simulink model "Rotational_to_linear"  (R2019a)
settings: Solver=VariableStepAuto  StartTime=0.0  StopTime=10  RelTol=1e-3
undefined symbols (not defined in the file): k_A, k_B, sigma_A, sigma_B
libraries: simulink x4
settings Model: Creator=wsimpson  LastModifiedBy=wsimpson

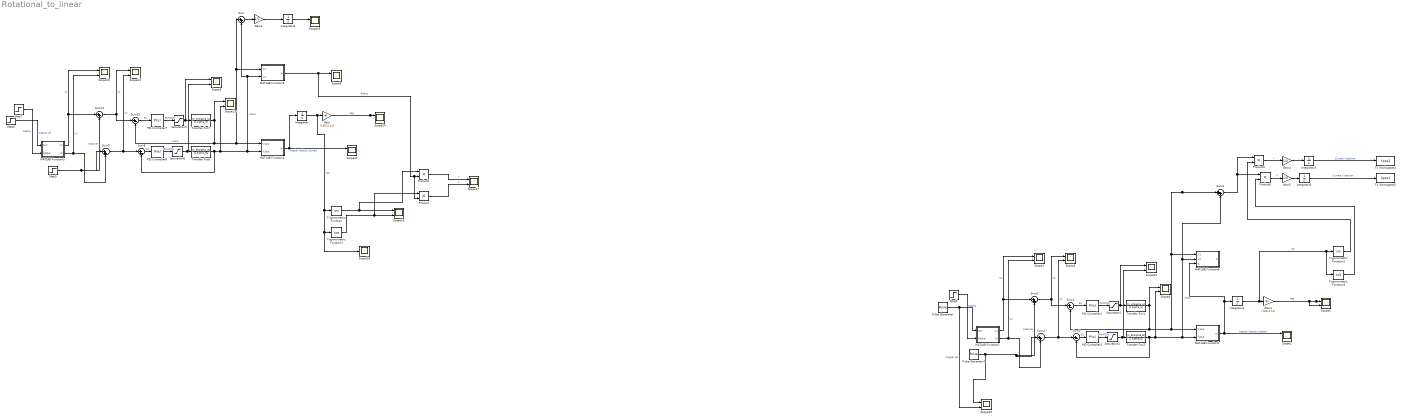
== system Rotational_to_linear ==
  Gain : Gain  Gain=(180/3.14)
  Gain1 : Gain  Gain=(180/3.14)
  Gain2 : Gain  Gain=1/2
  Gain4 : Gain  Gain=1/2
  Gain5 : Gain  Gain=1/2
  Integrator{,1,3..5} (5 alike) : Integrator
  MATLAB Function1 : MATLAB Function  TreatAsAtomicUnit=on
  MATLAB Function2 : MATLAB Function  TreatAsAtomicUnit=on
  MATLAB Function3 : MATLAB Function  TreatAsAtomicUnit=on
  MATLAB Function4 : MATLAB Function  TreatAsAtomicUnit=on
  MATLAB Function5 : MATLAB Function  TreatAsAtomicUnit=on
  MATLAB Function6 : MATLAB Function  TreatAsAtomicUnit=on
  PID Controller1 : simulink/Continuous/PID Controller  Controller=PI  Form=Parallel  TimeDomain=Continuous-time  SampleTime=-1  IntegratorMethod=Forward Euler  FilterMethod=Forward Euler  ControllerParametersSource=internal  P=46.2979731521748  I=461.590792327183  D=0  UseFilter=on  N=100  TunerSelectOption=Transfer Function Based (PID Tuner App)  InitialConditionSource=internal  InitialConditionForIntegrator=0  InitialConditionForFilter=0  DifferentiatorICPrevScaledInput=0  ExternalReset=none  TrackingMode=off  Kt=1  LimitOutput=off  UpperSaturationLimit=inf  LowerSaturationLimit=-inf  LinearizeAsGain=on  AntiWindupMode=none  Kb=1  POutMin=[]  POutMax=[]  IOutMin=[]  IOutMax=[]  DOutMin=[]  DOutMax=[]  NOutMin=[]  NOutMax=[]  SumOutMin=[]  SumOutMax=[]  SaturationOutMin=[]  SaturationOutMax=[]  PParamMin=[]  PParamMax=[]  IParamMin=[]  IParamMax=[]  DParamMin=[]  DParamMax=[]  NParamMin=[]  NParamMax=[]  KbParamMin=[]  KbParamMax=[]  KtParamMin=[]  KtParamMax=[]  KbOutMin=[]  KbOutMax=[]  KtOutMin=[]  KtOutMax=[]  IntegratorOutMin=[]  IntegratorOutMax=[]  FilterOutMin=[]  FilterOutMax=[]  SumI1OutMin=[]  SumI1OutMax=[]  SumI2OutMin=[]  SumI2OutMax=[]  SumI3OutMin=[]  SumI3OutMax=[]  SumI4OutMin=[]  SumI4OutMax=[]  SumDOutMin=[]  SumDOutMax=[]  DifferentiatorOutMin=[]  DifferentiatorOutMax=[]  FilterDiffOutCoefMin=[]  FilterDiffOutCoefMax=[]  ReciprocalOutMin=[]  ReciprocalOutMax=[]  SumDenOutMin=[]  SumDenOutMax=[]  SumNumOutMin=[]  SumNumOutMax=[]  DivideOutMin=[]  DivideOutMax=[]  IntegratorContinuousStateAttributes=''  IntegratorStateMustResolveToSignalObject=off  IntegratorRTWStateStorageClass=Auto  FilterContinuousStateAttributes=''  FilterStateMustResolveToSignalObject=off  FilterRTWStateStorageClass=Auto  ParallelPVariant=InternalParameters  IdealPVariant=Disabled  IVariant=InternalParameters  DVariant=Disabled  IntegratorVariant=Continuous  SatVariant=Disabled  AWVariant=Passthrough  PCopyVariant=Disabled  TRVariant=Disabled  FdbkBlocksVariant=Forward  IdealPFdbkVariant=Disabled  SatFdbkVariant=Disabled  DerivativeFilterVariant=Disabled  NVariant=Disabled  NCopyVariant=Disabled_SignalSpec  FilterICVariant=Disabled  IntegratorICVariant=InternalICs  ExternalResetVariant=Disabled  TRSumVariant=Passthrough  SumFdbkVariant=Disabled  SumVariant=Sum_PI
  PID Controller2 : simulink/Continuous/PID Controller  Controller=PI  Form=Parallel  TimeDomain=Continuous-time  SampleTime=-1  IntegratorMethod=Forward Euler  FilterMethod=Forward Euler  ControllerParametersSource=internal  P=46.6050777553275  I=515.918210751475  D=0  UseFilter=on  N=100  TunerSelectOption=Transfer Function Based (PID Tuner App)  InitialConditionSource=internal  InitialConditionForIntegrator=0  InitialConditionForFilter=0  DifferentiatorICPrevScaledInput=0  ExternalReset=none  TrackingMode=off  Kt=1  LimitOutput=off  UpperSaturationLimit=inf  LowerSaturationLimit=-inf  LinearizeAsGain=on  AntiWindupMode=none  Kb=1  POutMin=[]  POutMax=[]  IOutMin=[]  IOutMax=[]  DOutMin=[]  DOutMax=[]  NOutMin=[]  NOutMax=[]  SumOutMin=[]  SumOutMax=[]  SaturationOutMin=[]  SaturationOutMax=[]  PParamMin=[]  PParamMax=[]  IParamMin=[]  IParamMax=[]  DParamMin=[]  DParamMax=[]  NParamMin=[]  NParamMax=[]  KbParamMin=[]  KbParamMax=[]  KtParamMin=[]  KtParamMax=[]  KbOutMin=[]  KbOutMax=[]  KtOutMin=[]  KtOutMax=[]  IntegratorOutMin=[]  IntegratorOutMax=[]  FilterOutMin=[]  FilterOutMax=[]  SumI1OutMin=[]  SumI1OutMax=[]  SumI2OutMin=[]  SumI2OutMax=[]  SumI3OutMin=[]  SumI3OutMax=[]  SumI4OutMin=[]  SumI4OutMax=[]  SumDOutMin=[]  SumDOutMax=[]  DifferentiatorOutMin=[]  DifferentiatorOutMax=[]  FilterDiffOutCoefMin=[]  FilterDiffOutCoefMax=[]  ReciprocalOutMin=[]  ReciprocalOutMax=[]  SumDenOutMin=[]  SumDenOutMax=[]  SumNumOutMin=[]  SumNumOutMax=[]  DivideOutMin=[]  DivideOutMax=[]  IntegratorContinuousStateAttributes=''  IntegratorStateMustResolveToSignalObject=off  IntegratorRTWStateStorageClass=Auto  FilterContinuousStateAttributes=''  FilterStateMustResolveToSignalObject=off  FilterRTWStateStorageClass=Auto  ParallelPVariant=InternalParameters  IdealPVariant=Disabled  IVariant=InternalParameters  DVariant=Disabled  IntegratorVariant=Continuous  SatVariant=Disabled  AWVariant=Passthrough  PCopyVariant=Disabled  TRVariant=Disabled  FdbkBlocksVariant=Forward  IdealPFdbkVariant=Disabled  SatFdbkVariant=Disabled  DerivativeFilterVariant=Disabled  NVariant=Disabled  NCopyVariant=Disabled_SignalSpec  FilterICVariant=Disabled  IntegratorICVariant=InternalICs  ExternalResetVariant=Disabled  TRSumVariant=Passthrough  SumFdbkVariant=Disabled  SumVariant=Sum_PI
  PID Controller7 : simulink/Continuous/PID Controller  Controller=PI  Form=Parallel  TimeDomain=Continuous-time  SampleTime=-1  IntegratorMethod=Forward Euler  FilterMethod=Forward Euler  ControllerParametersSource=internal  P=46.2979731521748  I=461.590792327183  D=0  UseFilter=on  N=100  TunerSelectOption=Transfer Function Based (PID Tuner App)  InitialConditionSource=internal  InitialConditionForIntegrator=0  InitialConditionForFilter=0  DifferentiatorICPrevScaledInput=0  ExternalReset=none  TrackingMode=off  Kt=1  LimitOutput=off  UpperSaturationLimit=inf  LowerSaturationLimit=-inf  LinearizeAsGain=on  AntiWindupMode=none  Kb=1  POutMin=[]  POutMax=[]  IOutMin=[]  IOutMax=[]  DOutMin=[]  DOutMax=[]  NOutMin=[]  NOutMax=[]  SumOutMin=[]  SumOutMax=[]  SaturationOutMin=[]  SaturationOutMax=[]  PParamMin=[]  PParamMax=[]  IParamMin=[]  IParamMax=[]  DParamMin=[]  DParamMax=[]  NParamMin=[]  NParamMax=[]  KbParamMin=[]  KbParamMax=[]  KtParamMin=[]  KtParamMax=[]  KbOutMin=[]  KbOutMax=[]  KtOutMin=[]  KtOutMax=[]  IntegratorOutMin=[]  IntegratorOutMax=[]  FilterOutMin=[]  FilterOutMax=[]  SumI1OutMin=[]  SumI1OutMax=[]  SumI2OutMin=[]  SumI2OutMax=[]  SumI3OutMin=[]  SumI3OutMax=[]  SumI4OutMin=[]  SumI4OutMax=[]  SumDOutMin=[]  SumDOutMax=[]  DifferentiatorOutMin=[]  DifferentiatorOutMax=[]  FilterDiffOutCoefMin=[]  FilterDiffOutCoefMax=[]  ReciprocalOutMin=[]  ReciprocalOutMax=[]  SumDenOutMin=[]  SumDenOutMax=[]  SumNumOutMin=[]  SumNumOutMax=[]  DivideOutMin=[]  DivideOutMax=[]  IntegratorContinuousStateAttributes=''  IntegratorStateMustResolveToSignalObject=off  IntegratorRTWStateStorageClass=Auto  FilterContinuousStateAttributes=''  FilterStateMustResolveToSignalObject=off  FilterRTWStateStorageClass=Auto  ParallelPVariant=InternalParameters  IdealPVariant=Disabled  IVariant=InternalParameters  DVariant=Disabled  IntegratorVariant=Continuous  SatVariant=Disabled  AWVariant=Passthrough  PCopyVariant=Disabled  TRVariant=Disabled  FdbkBlocksVariant=Forward  IdealPFdbkVariant=Disabled  SatFdbkVariant=Disabled  DerivativeFilterVariant=Disabled  NVariant=Disabled  NCopyVariant=Disabled_SignalSpec  FilterICVariant=Disabled  IntegratorICVariant=InternalICs  ExternalResetVariant=Disabled  TRSumVariant=Passthrough  SumFdbkVariant=Disabled  SumVariant=Sum_PI
  PID Controller8 : simulink/Continuous/PID Controller  Controller=PI  Form=Parallel  TimeDomain=Continuous-time  SampleTime=-1  IntegratorMethod=Forward Euler  FilterMethod=Forward Euler  ControllerParametersSource=internal  P=46.6050777553275  I=515.918210751475  D=0  UseFilter=on  N=100  TunerSelectOption=Transfer Function Based (PID Tuner App)  InitialConditionSource=internal  InitialConditionForIntegrator=0  InitialConditionForFilter=0  DifferentiatorICPrevScaledInput=0  ExternalReset=none  TrackingMode=off  Kt=1  LimitOutput=off  UpperSaturationLimit=inf  LowerSaturationLimit=-inf  LinearizeAsGain=on  AntiWindupMode=none  Kb=1  POutMin=[]  POutMax=[]  IOutMin=[]  IOutMax=[]  DOutMin=[]  DOutMax=[]  NOutMin=[]  NOutMax=[]  SumOutMin=[]  SumOutMax=[]  SaturationOutMin=[]  SaturationOutMax=[]  PParamMin=[]  PParamMax=[]  IParamMin=[]  IParamMax=[]  DParamMin=[]  DParamMax=[]  NParamMin=[]  NParamMax=[]  KbParamMin=[]  KbParamMax=[]  KtParamMin=[]  KtParamMax=[]  KbOutMin=[]  KbOutMax=[]  KtOutMin=[]  KtOutMax=[]  IntegratorOutMin=[]  IntegratorOutMax=[]  FilterOutMin=[]  FilterOutMax=[]  SumI1OutMin=[]  SumI1OutMax=[]  SumI2OutMin=[]  SumI2OutMax=[]  SumI3OutMin=[]  SumI3OutMax=[]  SumI4OutMin=[]  SumI4OutMax=[]  SumDOutMin=[]  SumDOutMax=[]  DifferentiatorOutMin=[]  DifferentiatorOutMax=[]  FilterDiffOutCoefMin=[]  FilterDiffOutCoefMax=[]  ReciprocalOutMin=[]  ReciprocalOutMax=[]  SumDenOutMin=[]  SumDenOutMax=[]  SumNumOutMin=[]  SumNumOutMax=[]  DivideOutMin=[]  DivideOutMax=[]  IntegratorContinuousStateAttributes=''  IntegratorStateMustResolveToSignalObject=off  IntegratorRTWStateStorageClass=Auto  FilterContinuousStateAttributes=''  FilterStateMustResolveToSignalObject=off  FilterRTWStateStorageClass=Auto  ParallelPVariant=InternalParameters  IdealPVariant=Disabled  IVariant=InternalParameters  DVariant=Disabled  IntegratorVariant=Continuous  SatVariant=Disabled  AWVariant=Passthrough  PCopyVariant=Disabled  TRVariant=Disabled  FdbkBlocksVariant=Forward  IdealPFdbkVariant=Disabled  SatFdbkVariant=Disabled  DerivativeFilterVariant=Disabled  NVariant=Disabled  NCopyVariant=Disabled_SignalSpec  FilterICVariant=Disabled  IntegratorICVariant=InternalICs  ExternalResetVariant=Disabled  TRSumVariant=Passthrough  SumFdbkVariant=Disabled  SumVariant=Sum_PI
  Product{,1,4..5} (4 alike) : Product
  Pulse Generator : DiscretePulseGenerator  PulseType=Time based  Amplitude=1.25  Period=10  PulseWidth=50
  Pulse Generator1 : DiscretePulseGenerator  PulseType=Time based  Amplitude=1.5  Period=10  PulseWidth=50  PhaseDelay=5
  Saturation{1..2,5..6} (4 alike) : Saturate  UpperLimit=300  LowerLimit=-300
  Scope{1..5,8..17,19,22} (17 alike) : Scope  NumInputPorts=2
  Scope18 : Scope
  Step3 : Step  Time=0  SampleTime=0
  Step5 : Step  Time=0  After=0  SampleTime=0
  Step6 : Step  Time=0  After=1.25  SampleTime=0
  Step7 : Step  Time=0  SampleTime=0
  Sum{,2,4,6,9,11} (6 alike) : Sum  Inputs=|++
  Sum{1,3,8,10} (4 alike) : Sum  Inputs=|+-
  To Workspace3 : ToWorkspace  VariableName=Xpos1  SaveFormat=Timeseries  SampleTime=-1
  To Workspace4 : ToWorkspace  VariableName=Ypos1  SaveFormat=Timeseries  SampleTime=-1
  Transfer Fcn1 : TransferFcn  Numerator=[k_A*sigma_A]  Denominator=[1 sigma_A]
  Transfer Fcn2 : TransferFcn  Numerator=[k_B*sigma_B]  Denominator=[1 sigma_B]
  Transfer Fcn7 : TransferFcn  Numerator=[k_A*sigma_A]  Denominator=[1 sigma_A]
  Transfer Fcn8 : TransferFcn  Numerator=[k_B*sigma_B]  Denominator=[1 sigma_B]
  Trigonometric Function : Trigonometry
  Trigonometric Function1 : Trigonometry  Operator=cos
  Trigonometric Function2 : Trigonometry
  Trigonometric Function3 : Trigonometry  Operator=cos
  wires:
  Saturation6/1 -> Scope9/2, Transfer Fcn8/1
  Saturation5/1 -> Scope9/1, Transfer Fcn7/1
  MATLAB Function3/2(V2) -> Scope10/2, Sum9/2  "V2"
  Transfer Fcn7/1 -> Scope13/1, Sum10/2, Sum/1, MATLAB Function5/1(V1), MATLAB Function4/1(V1out)  "V1out"
  Transfer Fcn8/1 -> Scope13/2, Sum/2, MATLAB Function5/2(V2), MATLAB Function4/2(V2out), Sum8/2  "V2out"
  Step5/1 -> Sum11/2, Sum9/1  "linearVel"
  Sum11/1 -> Sum10/1, Scope12/1  "V1"
  Sum8/1 -> PID Controller8/1  "E2"
  PID Controller8/1 -> Saturation6/1  "PWMCNt"
  Sum9/1 -> Scope12/2, Sum8/1  "V2"
  PID Controller7/1 -> Saturation5/1  "PWMCNt"
  Sum10/1 -> PID Controller7/1  "E1"
  MATLAB Function5/1(R) -> Scope8/1, Product/2, Product1/2  "Radius"
  MATLAB Function4/1(W) -> Scope11/1, Integrator/1  "Angular Velocity System"
  MATLAB Function3/1(V1) -> Scope10/1, Sum11/1  "V1"
  Step7/1 -> MATLAB Function3/2(Radius)  "Radius"
  Integrator/1 -> Scope18/1, Trigonometric Function1/1, Trigonometric Function/1, Gain/1  "rad"
  Step6/1 -> MATLAB Function3/1(Wrc)  "Angular vel"
  Trigonometric Function/1 -> Product1/1, Scope16/1
  Gain/1 -> Scope14/1  "deg"
  Trigonometric Function1/1 -> Product/1, Scope16/2
  Product1/1 -> Scope17/1  "Y"
  Product/1 -> Scope17/2  "X"
  Sum4/1 -> Scope3/2, Sum3/1  "V2"
  PID Controller2/1 -> Saturation2/1  "PWMCNt"
  Saturation2/1 -> Scope22/2, Transfer Fcn2/1
  MATLAB Function1/2(V2) -> Scope1/2, Sum4/2  "V2"
  Sum2/1 -> Sum1/1, Scope3/1  "V1"
  PID Controller1/1 -> Saturation1/1  "PWMCNt"
  Sum1/1 -> PID Controller1/1  "E1"
  Saturation1/1 -> Scope22/1, Transfer Fcn1/1
  Sum3/1 -> PID Controller2/1  "E2"
  Pulse Generator/1 -> Scope19/2, MATLAB Function1/1(Wrc)  "Angular vel"
  MATLAB Function1/1(V1) -> Scope1/1, Sum2/1  "V1"
  Integrator1/1 -> Trigonometric Function3/1, Trigonometric Function2/1, Gain1/1  "rad"
  Gain1/1 -> Scope5/2, Scope5/1  "deg"
  Pulse Generator1/1 -> Scope19/1, Sum2/2, Sum4/1  "linearVel"
  Transfer Fcn2/1 -> Scope4/2, Sum6/2, MATLAB Function6/2(V2), MATLAB Function2/2(V2out), Sum3/2  "V2out"
  Trigonometric Function2/1 -> Product4/2
  Transfer Fcn1/1 -> Scope4/1, Sum1/2, Sum6/1, MATLAB Function6/1(V1), MATLAB Function2/1(V1out)
  Step3/1 -> MATLAB Function1/2(Radius)  "Radius"
  MATLAB Function2/1(W) -> MATLAB Function6/3(w), Integrator1/1, Scope2/1  "Angular Velocity System"
  Sum/1 -> Gain2/1
  Gain2/1 -> Integrator4/1
  Integrator4/1 -> Scope15/1
  Trigonometric Function3/1 -> Product5/2
  Sum6/1 -> Product5/1, Product4/1
  Product4/1 -> Gain4/1  "Y"
  Product5/1 -> Gain5/1  "X"
  Gain4/1 -> Integrator3/1
  Gain5/1 -> Integrator5/1
  Integrator3/1 -> To Workspace4/1  "Current Y position"
  Integrator5/1 -> To Workspace3/1  "Current X position"

== matlab function Rotational_to_linear/MATLAB Function1 ==
  data: Wrc input; V1 output; V2 output; Radius input
function [V1,V2] = fcn(Wrc,Radius)

L=13.125/12;
if Radius > 0
V1=Wrc*(Radius+L/2);
V2=Wrc*(Radius-L/2);
else
V2=Wrc*(Radius+L/2);
V1=Wrc*(Radius-L/2);
end

== matlab function Rotational_to_linear/MATLAB Function2 ==
  data: V1out input; W output; V2out input
 function W = fcn(V1out,V2out)

d=13.125/12;
W = (V1out-V2out)/(d);

== matlab function Rotational_to_linear/MATLAB Function6 ==
  data: V1 input; R output; V2 input; w input
function R  = fcn(V1,V2,w)

    Vl1=0;
    Vl2=0;
    l=13.15/12;
    R = (l/2)*((V2+V1)/(V1-V2));

== matlab function Rotational_to_linear/MATLAB Function3 ==
  data: Wrc input; V1 output; V2 output; Radius input
function [V1,V2] = fcn(Wrc,Radius)

L=13.125/12;
if Radius > 0
V1=Wrc*(Radius+L/2);
V2=Wrc*(Radius-L/2);
else
V2=Wrc*(Radius+L/2);
V1=Wrc*(Radius-L/2);
end

== matlab function Rotational_to_linear/MATLAB Function4 ==
  data: V1out input; W output; V2out input
 function W = fcn(V1out,V2out)

d=13.125/12;
W = (V1out-V2out)/(d);

== matlab function Rotational_to_linear/MATLAB Function5 ==
  data: V1 input; R output; V2 input
function R = fcn(V1,V2)

l=13.125/12;
R = (l/2)*((V2+V1)/(V1-V2));
